simulink model "statek"  (Simulink 7.1)
settings: Solver=ode45  StartTime=0.0  StopTime=1000.0  RelTol=1e-3
settings Model: Creator=M.Plucinski  ModifiedByFormat=M.Plucinski  LastModifiedBy=M.Plucinski

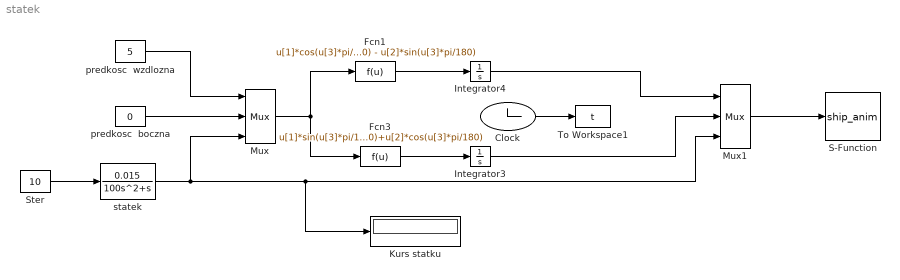
== system statek ==
  Clock : Clock
      settings: Decimation=10
  Fcn1 : Fcn  Expr=u[1]*cos(u[3]*pi/180) - u[2]*sin(u[3]*pi/180)
  Fcn3 : Fcn  Expr=u[1]*sin(u[3]*pi/180)+u[2]*cos(u[3]*pi/180)
  Integrator3 : Integrator
  Integrator4 : Integrator
  Kurs statku : Display
  Mux : Mux  Inputs=3
  Mux1 : Mux  Inputs=3
  S-Function : S-Function  FunctionName=ship_anim  Parameters=1  EnableBusSupport=off
  Ster : Constant  Value=10  OutDataType=sfix(16)  OutScaling=2^0
  To Workspace1 : ToWorkspace  VariableName=t  SampleTime=0.1  SaveFormat=Array
  predkosc  boczna : Constant  Value=0  OutDataType=sfix(16)  OutScaling=2^0
  predkosc  wzdlozna : Constant  Value=5  OutDataType=sfix(16)  OutScaling=2^0
  statek : TransferFcn  Numerator=[0.015]  Denominator=[100 1 0]  ContinuousStateAttributes='ship'
  wires:
  Mux1/1 -> S-Function/1
  Ster/1 -> statek/1
  Fcn3/1 -> Integrator3/1
  predkosc  boczna/1 -> Mux/2
  Fcn1/1 -> Integrator4/1
  Mux/1 -> Fcn1/1, Fcn3/1
  Clock/1 -> To Workspace1/1
  statek/1 -> Mux/3, Mux1/3, Kurs statku/1
  predkosc  wzdlozna/1 -> Mux/1
  Integrator4/1 -> Mux1/1
  Integrator3/1 -> Mux1/2
